simulink model "ServoAmira"  (R2023b)
settings: Solver=ode23  StartTime=0.0  StopTime=10  MaxStep=0.1  RelTol=1e-3  EnableMultiTasking=on
InitFcn:
  | g = 9.81; %gravitational constant
  | 
  | 
  | % showVR = 1; %show VR world
  | % ig_init = 0; %initial condition
  | % im_init = 0; %initial condition
  | % omega_init = 0; %initial condition
  | % phi_init = 0; %initial condition
values from neighbouring files (symbols this model uses):
  b = 2.1E-5    (= 2.1e-05)    [motor_constants.m]
  bg = 1E-5    (= 1e-05)    [motor_constants.m]
  J = 1.8E-5    (= 1.8e-05)    [motor_constants.m]
  Jg = J / 7    (= 2.57142857143e-06)    [motor_constants.m]
  ke = 0.05    [motor_constants.m]
  keg = 0.09    [motor_constants.m]
  km = 0.18    [motor_constants.m]
  kmg = 0.12    [motor_constants.m]
  L = 0.3    [motor_constants.m]
  Lg = 0.1    [motor_constants.m]
  R = 5    [motor_constants.m]
  Rg = 1    [motor_constants.m]
libraries: vrlib x4, slpidlib x2, simulink x1
CloseFcn:
  | vrclose all;
  | clear figureVR worldVR;
settings Model: Creator=Luky  LastModifiedBy=Lenovo
settings DataIOCC: LimitDataPoints=on  SaveFormat=Array  SignalLoggingSaveFormat=ModelDataLogs  ReturnWorkspaceOutputs=off
settings OptimizationCC: ExpressionDepthLimit=2147483647  InitFltsAndDblsToZero=on  LifeSpan=inf
settings DebuggingCC: SaveWithParameterizedLinksMsg=none  UnderspecifiedInitializationDetection=Classic  MergeDetectMultiDrivingBlocksExec=none  SolverPrmCheckMsg=warning  FcnCallInpInsideContextMsg=warning  UnconnectedInputMsg=warning  UnconnectedOutputMsg=warning  UnconnectedLineMsg=warning  StateNameClashWarn=warning  SFUnexpectedBacktrackingDiag=warning  SFNoUnconditionalDefaultTransitionDiag=warning  SFExecutionAtInitializationDiag=none  ArithmeticOperatorsInVariantConditions=warning
settings HardwareCC: ProdBitPerPointer=32  ProdBitPerSizeT=32  ProdBitPerPtrDiffT=32  ProdLargestAtomicFloat=None  ProdIntDivRoundTo=Undefined  ProdEndianess=Unspecified  ProdWordSize=32  ProdHWDeviceType=32-bit Generic
settings ModelReferenceCC: PropagateSignalLabelsOutOfModel=off
settings SFSimCC: SimUseLocalCustomCode=off  CustomCodeUndefinedFunction=UseInterfaceOnly
settings RTWCC: RTWUseLocalCustomCode=off
settings CodeAppCC: StateflowObjectComments=on
settings GRTTargetCC: TargetLangStandard=C89/C90 (ANSI)  CombineOutputUpdateFcns=off  GRTInterface=on
settings ConfigComp: CovMetricSettings=dw  CovSaveCumulativeToWorkspaceVar=on  CovSaveSingleToWorkspaceVar=on  CovExternalEMLEnable=off

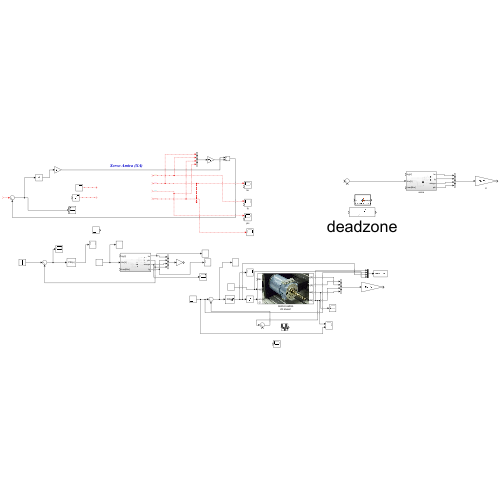
[thumbnail: Simulink's stored preview of the top-level diagram]
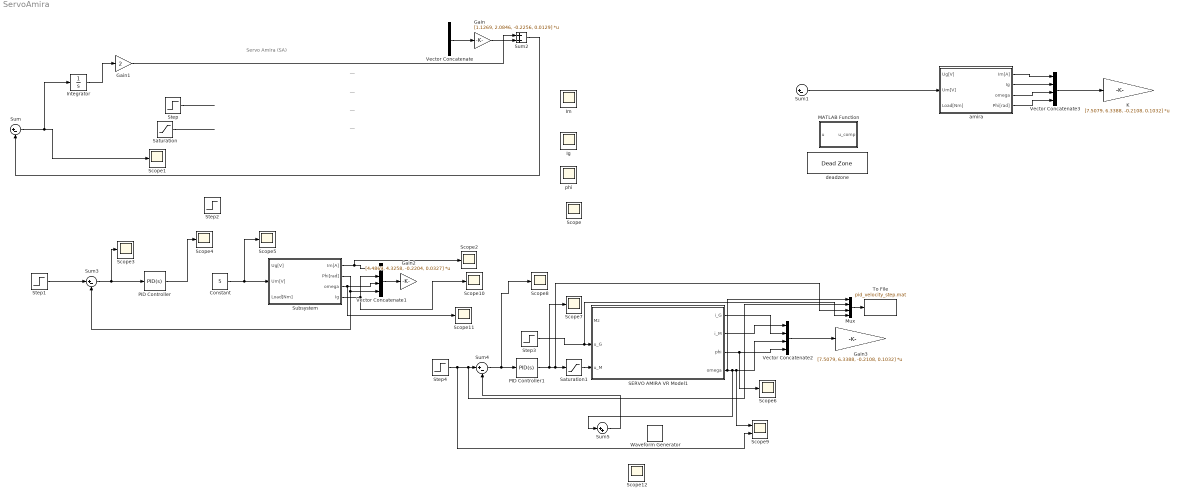
== system ServoAmira ==
  note: Servo Amira (SA)
  note: __
  note: __
  note: __
  note: __
  Constant : Constant  Value=5
  Gain : Gain  Gain=[1.1269, 2.0846, -0.2256, 0.0129]  Multiplication=Matrix(K*u)
  Gain1 : Gain  Gain=2
  Gain2 : Gain  Gain=[4.4869, 4.3258, -0.2204, 0.0327]  Multiplication=Matrix(K*u)
  Gain3 : Gain  Gain=[7.5079, 6.3388, -0.2108, 0.1032]  Multiplication=Matrix(K*u)
  Ig : Scope  NumInputPorts=2
  Im : Scope  NumInputPorts=2
  Integrator : Integrator
  K : Gain  Gain=[7.5079, 6.3388, -0.2108, 0.1032]  Multiplication=Matrix(K*u)
  MATLAB Function : MATLAB Function  TreatAsAtomicUnit=on
  Mux : Mux
  PID Controller : slpidlib/PID Controller  Controller=PID  Form=Parallel  TimeDomain=Continuous-time  UseExternalTs=off  SampleTime=-1  IntegratorMethod=Forward Euler  FilterMethod=Forward Euler  ControllerParametersSource=internal  P=0.1  I=0.1  UseKiTs=off  D=0  N=100  UseFilter=on  TunerSelectOption=Transfer Function Based (PID Tuner App)  InitialConditionSource=internal  InitialConditionForIntegrator=0  InitialConditionForFilter=0  DifferentiatorICPrevScaledInput=0  ExternalReset=none  TrackingMode=off  Kt=1  LimitOutput=off  SatLimitsSource=internal  UpperSaturationLimit=inf  LowerSaturationLimit=-inf  LinearizeAsGain=on  AntiWindupMode=none  Kb=1  LimitIntegrator=off  UpperIntegratorSaturationLimit=inf  LowerIntegratorSaturationLimit=-inf  POutMin=[]  POutMax=[]  IOutMin=[]  IOutMax=[]  DOutMin=[]  DOutMax=[]  NOutMin=[]  NOutMax=[]  SumOutMin=[]  SumOutMax=[]  SaturationOutMin=[]  SaturationOutMax=[]  PParamMin=[]  PParamMax=[]  IParamMin=[]  IParamMax=[]  DParamMin=[]  DParamMax=[]  NParamMin=[]  NParamMax=[]  KbParamMin=[]  KbParamMax=[]  KtParamMin=[]  KtParamMax=[]  KbOutMin=[]  KbOutMax=[]  KtOutMin=[]  KtOutMax=[]  IntegratorOutMin=[]  IntegratorOutMax=[]  FilterOutMin=[]  FilterOutMax=[]  SumI1OutMin=[]  SumI1OutMax=[]  SumI2OutMin=[]  SumI2OutMax=[]  SumI3OutMin=[]  SumI3OutMax=[]  SumI4OutMin=[]  SumI4OutMax=[]  SumDOutMin=[]  SumDOutMax=[]  DifferentiatorOutMin=[]  DifferentiatorOutMax=[]  FilterDiffOutCoefMin=[]  FilterDiffOutCoefMax=[]  ReciprocalOutMin=[]  ReciprocalOutMax=[]  SumDenOutMin=[]  SumDenOutMax=[]  SumNumOutMin=[]  SumNumOutMax=[]  DivideOutMin=[]  DivideOutMax=[]  UdiffTsProdOutMin=[]  UdiffTsProdOutMax=[]  NTsProdOutMin=[]  NTsProdOutMax=[]  UintegralTsProdOutMin=[]  UintegralTsProdOutMax=[]  UngainTsProdOutMin=[]  UngainTsProdOutMax=[]  ClampingZeroOutDataTypeStr=Inherit: Inherit via back propagation  ClampingZeroOutMin=[]  ClampingZeroOutMax=[]  FilterDenConstantOutDataTypeStr=Inherit: Inherit via back propagation  FilterDenConstantOutMin=[]  FilterDenConstantOutMax=[]  PCopyOutDataTypeStr=Inherit: Inherit via back propagation  PCopyOutMin=[]  PCopyOutMax=[]  NCopyOutDataTypeStr=Inherit: Inherit via back propagation  NCopyOutMin=[]  NCopyOutMax=[]  IntegratorContinuousStateAttributes=''  IntegratorStateMustResolveToSignalObject=off  IntegratorRTWStateStorageClass=Auto  FilterContinuousStateAttributes=''  FilterStateMustResolveToSignalObject=off  FilterRTWStateStorageClass=Auto  ParallelPVariant=InternalParameters  IdealPVariant=Disabled  IVariant=InternalParameters  DVariant=InternalParameters  IntegratorVariant=Continuous  SatVariant=Disabled  AWVariant=Passthrough  PCopyVariant=Disabled  TRVariant=Disabled  FdbkBlocksVariant=Forward  IdealPFdbkVariant=Disabled  SatFdbkVariant=Disabled  DerivativeFilterVariant=ContFilter  NVariant=InternalParameters  NCopyVariant=Disabled  FilterICVariant=InternalICsFilter  IntegratorICVariant=InternalICs  ExternalResetVariant=Disabled  TRSumVariant=Passthrough  SumFdbkVariant=Disabled  SumVariant=Sum_PID  TsampFilterVariant=InternalTs  TsampNgainVariant=Passthrough  TsampIntegralVariant=Disabled_SignalSpec  ExternalSaturationOutDataTypeStr=Inherit: Same as second input
  PID Controller1 : slpidlib/PID Controller  Controller=PID  Form=Parallel  TimeDomain=Continuous-time  UseExternalTs=off  SampleTime=-1  IntegratorMethod=Forward Euler  FilterMethod=Forward Euler  ControllerParametersSource=internal  P=0.7401  I=2.6831  UseKiTs=off  D=0.0462  N=150  UseFilter=on  TunerSelectOption=Transfer Function Based (PID Tuner App)  InitialConditionSource=internal  InitialConditionForIntegrator=0  InitialConditionForFilter=0  DifferentiatorICPrevScaledInput=0  ExternalReset=none  TrackingMode=off  Kt=1  LimitOutput=on  SatLimitsSource=internal  UpperSaturationLimit=10  LowerSaturationLimit=-9.9  LinearizeAsGain=on  AntiWindupMode=back-calculation  Kb=1  LimitIntegrator=off  UpperIntegratorSaturationLimit=inf  LowerIntegratorSaturationLimit=-inf  POutMin=[]  POutMax=[]  IOutMin=[]  IOutMax=[]  DOutMin=[]  DOutMax=[]  NOutMin=[]  NOutMax=[]  SumOutMin=[]  SumOutMax=[]  SaturationOutMin=[]  SaturationOutMax=[]  PParamMin=[]  PParamMax=[]  IParamMin=[]  IParamMax=[]  DParamMin=[]  DParamMax=[]  NParamMin=[]  NParamMax=[]  KbParamMin=[]  KbParamMax=[]  KtParamMin=[]  KtParamMax=[]  KbOutMin=[]  KbOutMax=[]  KtOutMin=[]  KtOutMax=[]  IntegratorOutMin=[]  IntegratorOutMax=[]  FilterOutMin=[]  FilterOutMax=[]  SumI1OutMin=[]  SumI1OutMax=[]  SumI2OutMin=[]  SumI2OutMax=[]  SumI3OutMin=[]  SumI3OutMax=[]  SumI4OutMin=[]  SumI4OutMax=[]  SumDOutMin=[]  SumDOutMax=[]  DifferentiatorOutMin=[]  DifferentiatorOutMax=[]  FilterDiffOutCoefMin=[]  FilterDiffOutCoefMax=[]  ReciprocalOutMin=[]  ReciprocalOutMax=[]  SumDenOutMin=[]  SumDenOutMax=[]  SumNumOutMin=[]  SumNumOutMax=[]  DivideOutMin=[]  DivideOutMax=[]  UdiffTsProdOutMin=[]  UdiffTsProdOutMax=[]  NTsProdOutMin=[]  NTsProdOutMax=[]  UintegralTsProdOutMin=[]  UintegralTsProdOutMax=[]  UngainTsProdOutMin=[]  UngainTsProdOutMax=[]  ClampingZeroOutDataTypeStr=Inherit: Inherit via back propagation  ClampingZeroOutMin=[]  ClampingZeroOutMax=[]  FilterDenConstantOutDataTypeStr=Inherit: Inherit via back propagation  FilterDenConstantOutMin=[]  FilterDenConstantOutMax=[]  PCopyOutDataTypeStr=Inherit: Inherit via back propagation  PCopyOutMin=[]  PCopyOutMax=[]  NCopyOutDataTypeStr=Inherit: Inherit via back propagation  NCopyOutMin=[]  NCopyOutMax=[]  IntegratorContinuousStateAttributes=''  IntegratorStateMustResolveToSignalObject=off  IntegratorRTWStateStorageClass=Auto  FilterContinuousStateAttributes=''  FilterStateMustResolveToSignalObject=off  FilterRTWStateStorageClass=Auto  ParallelPVariant=InternalParameters  IdealPVariant=Disabled  IVariant=InternalParameters  DVariant=InternalParameters  IntegratorVariant=Continuous  SatVariant=Enabled  AWVariant=BackCalculation  PCopyVariant=Disabled  TRVariant=Disabled  FdbkBlocksVariant=Forward  IdealPFdbkVariant=Disabled  SatFdbkVariant=Disabled  DerivativeFilterVariant=ContFilter  NVariant=InternalParameters  NCopyVariant=Disabled  FilterICVariant=InternalICsFilter  IntegratorICVariant=InternalICs  ExternalResetVariant=Disabled  TRSumVariant=Passthrough  SumFdbkVariant=Disabled  SumVariant=Sum_PID  TsampFilterVariant=InternalTs  TsampNgainVariant=Passthrough  TsampIntegralVariant=Disabled_SignalSpec  ExternalSaturationOutDataTypeStr=Inherit: Same as second input
  SERVO AMIRA VR Model1 : Subsystem  mask(Servo Amira){showVR=on, sfcnParam1=0, sfcnParam2=0, sfcnParam3=0, sfcnParam4=0}
      mask prompts: showVR "Show VR?"; sfcnParam1 "Initial value of the current of the generator [A]"; sfcnParam2 "Initial value of the current of the motor  im [A]"; sfcnParam3 "Initial value of the angular speed  omega [rad/s]"; sfcnParam4 "Initial value of the angle of the motor shaft phi [rad]"
      mask help: Servo Amira - Virtual Reality
      mask Help:
      | Servo Amira - Virtual Reality <br><br>
      | 
      | 
      | This is a model of the direct current motor. Model is determined to demonstrate real system. It has two inputs, voltage and torgue. Outputs are rotational velocity of the shaft, current and position of the shaft. Virtual reality shows input and output values of the motor.
      | <br><br>
      | 
      | 
      | This is a virtual model of the Servo Amira laboratory model
      | in laboratory of automatic control theory&nbsp;26 (<a href="http://dce.felk.cvut.cz/lab26/" target="_blank">http://dce.felk.cvut.cz/lab26/</a>),
      | which consists of two identical motors (left and right) connected together with a very little flexible shaft. The left motor is used as a generator - it
      | can be used for simulation of a varying  moment of inertia. The right motor is used for control of the rotational speed of the servomechanism or
      | of the angle the motor shaft. <br><br>
      | 
      | There are two inputs and four outputs of the model. The inputs are voltages of the motors um [V] and ug [V] between -10 and 10 volts. Outputs
      | are the speed of the servomechanism omega [rad/s], the angle of the motor shaft phi [rad] and the currents of the motors im [A], ig [A].
      | More information can be found on the website <a href="http://dce.felk.cvut.cz/lab26/" target="_blank">http://dce.felk.cvut.cz/lab26/</a>.<br><br>
      | 
      | 
      | In the mask of the model, it can be set:
      | <ul>
      | <li>Initial value of the current of the generator</li>
      | <li>Initial value of the current of the motor</li>
      | <li>Initial value of the angular speed</li>
      | <li>Initial value of the angle of the motor shaft</li>
      | </ul><br><br>
      | 
      | 
      | Copyright: 2008,   Petr Prochazka, Jirka Roubal, Petr Husek.
      mask Callback showVR:
      | if strcmp('off',get_param(gcb,'showVR'))
      |     vrclose all;
      | else
      |     if exist('figureVR')==0
      |         figureVR = vrfigure;
      |     end
      |     if exist('worldVR')==0
      |         worldVR = vrworld('ServoAmira_VR.WRL');
      |     end
      | 	if isvalid(figureVR)==0
      |         open(worldVR);
      |         figureVR = vrfigure(worldVR,[650 80 550 350]);
      | 	end
      | end
      mask Display:
      | image(imread('ServoAmira_Image.jpg'))
      | port_label ('input',1,'Mz [Nm]')
      | port_label ('input',2,'ug [V]')
      | port_label ('input',3,'um [V]')
      | port_label ('output',1,'ig [A]')
      | port_label ('output',2,'im [A]')
      | port_label ('output',3,'phi [rad]')
      | port_label ('output',4,'omega [rad/s]')
  Saturation : Saturate  UpperLimit=10  LowerLimit=-9.9
  Saturation1 : Saturate  UpperLimit=10  LowerLimit=-9.9
  Scope{,2..8,10..12} (11 alike) : Scope
  Scope1 : Scope  NumInputPorts=3
  Scope9 : Scope  NumInputPorts=2
  Step : Step  Time=2  After=0  SampleTime=0
  Step1 : Step  After=10  SampleTime=0
  Step2 : Step  Time=3  After=0.1  SampleTime=0
  Step3 : Step  Time=4  After=2  SampleTime=0
  Step4 : Step  Time=0  After=20  SampleTime=0
  Subsystem : Subsystem
  Sum{,1,3..4} (4 alike) : Sum  Inputs=|+-
  Sum2 : Sum
  Sum5 : Sum  Inputs=|++
  To File : ToFile  Filename=pid_velocity_step.mat  SaveFormat=Timeseries
  Vector Concatenate{,1..3} (4 alike) : Concatenate  NumInputs=4
  Waveform Generator : simulink/Sources/Waveform Generator  OutMin=[]  OutMax=[]  OutDataTypeStr=double  SelectedSignal=1  Signals=gaussian(0, 0.25, 0)#  BlockNames=MultiportSwitch_1928104fab044be#MultiportSwitch_50f1443cd3b243a  SampleTime=0.05
  amira : Subsystem
  deadzone : DeadZone
  phi : Scope  NumInputPorts=2
  wires:
  ? -> Vector Concatenate/1, Im/1
  ? -> Vector Concatenate/2, Ig/1
  ? -> Vector Concatenate/4, phi/1
  ? -> Vector Concatenate/3, Scope/1
  Step/1 -> ?
  Vector Concatenate/1 -> Gain/1
  Saturation/1 -> ?
  Integrator/1 -> Gain1/1
  Gain1/1 -> Sum2/1
  Gain/1 -> Sum2/2
  Sum2/1 -> Sum/2
  Sum/1 -> Scope1/2, Integrator/1
  ? -> Sum/1
  Vector Concatenate1/1 -> Gain2/1
  Subsystem/1(Im[A]) -> Scope2/1, Vector Concatenate1/1
  Subsystem/4(Ig) -> Scope10/1, Vector Concatenate1/2
  Subsystem/3(omega) -> Scope11/1, Vector Concatenate1/3
  Subsystem/2(Phi[rad]) -> Sum3/2, Vector Concatenate1/4
  Constant/1 -> Scope5/1, Subsystem/2(Um[V])
  Step1/1 -> Sum3/1
  Sum3/1 -> PID Controller/1, Scope3/1
  PID Controller/1 -> Scope4/1
  Vector Concatenate2/1 -> Gain3/1
  SERVO AMIRA VR Model1/2("i_M ") -> Vector Concatenate2/1
  SERVO AMIRA VR Model1/1(i_G) -> Vector Concatenate2/2
  SERVO AMIRA VR Model1/3("phi ") -> Scope6/1, Vector Concatenate2/4
  Saturation1/1 -> SERVO AMIRA VR Model1/3(u_M)
  Mux/1 -> To File/1
  Sum4/1 -> PID Controller1/1, Scope8/1
  Vector Concatenate3/1 -> K/1
  amira/1(Im[A]) -> Vector Concatenate3/1
  amira/2(Ig) -> Vector Concatenate3/2
  amira/3(omega) -> Vector Concatenate3/3
  amira/4(Phi[rad]) -> Vector Concatenate3/4
  Sum1/1 -> amira/2(Um[V])
  PID Controller1/1 -> Scope7/1, Mux/3, Saturation1/1
  SERVO AMIRA VR Model1/4("omega ") -> Mux/1, Sum5/1, Scope9/1, Vector Concatenate2/3
  Step3/1 -> Mux/4, SERVO AMIRA VR Model1/2(u_G)
  Step4/1 -> Scope9/2, Mux/2, Sum4/1
  Sum5/1 -> Sum4/2

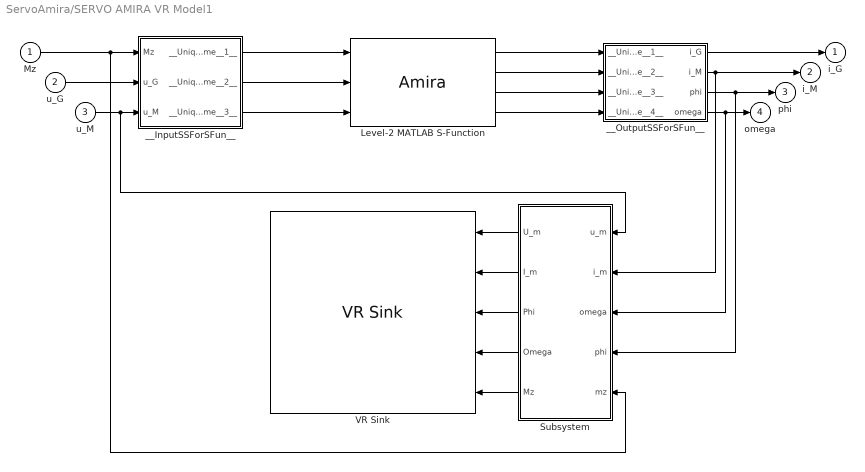
== system ServoAmira/SERVO AMIRA VR Model1 ==
  Mz : Inport
  u_G : Inport  Port=2
  u_M : Inport  Port=3
  Level-2 MATLAB S-Function : M-S-Function  FunctionName=Amira  Parameters=ig0 im0 omega0 psi0  mask{ig0=sfcnParam1, im0=sfcnParam2, omega0=sfcnParam3, psi0=sfcnParam4}
      mask prompts: ig0 "ig_init"; im0 "im_init"; omega0 "omega_init"; psi0 "psi_init"
      mask Display:
      | port_label('input',1,'Mz');
      | port_label('input',2,'u_G');
      | port_label('input',3,'u_M');
      | port_label('output',1,'i_G');
      | port_label('output',2,'i_M ');
      | port_label('output',3,'phi ');
      | port_label('output',4,'omega ');
  Subsystem : Subsystem
  VR Sink : vrlib/VR Sink  InstantiateOnLoad=on  SampleTime=0.1  ViewEnable=on  RemoteChange=off  RemoteView=on  FieldsWritten=show_u.translation.3.1.double#show_i.translation.3.1.double#fi.rotation.4.1.double#show_n.rotation.4.1.double#show_m.translation.3.1.double  WorldFileName=ServoAmira_VR.WRL  AutoView=off  VideoDimensions=[]  AllowVariableSize=off
  __InputSSForSFun__ : Subsystem
  __OutputSSForSFun__ : Subsystem
  i_G : Outport  OutDataTypeStr=double  PortDimensions=1  SampleTime=[-1 0]
  "i_M " : Outport  Port=2  OutDataTypeStr=double  PortDimensions=1  SampleTime=[-1 0]
  "phi " : Outport  Port=3  OutDataTypeStr=double  PortDimensions=1  SampleTime=[-1 0]
  "omega " : Outport  Port=4  OutDataTypeStr=double  PortDimensions=1  SampleTime=[-1 0]
  wires:
  Mz/1 -> __InputSSForSFun__/1(Mz), Subsystem/5(mz)
  u_G/1 -> __InputSSForSFun__/2(u_G)
  u_M/1 -> __InputSSForSFun__/3(u_M), Subsystem/1(u_m)
  __InputSSForSFun__/1(__UniqueOutportName__1__) -> Level-2 MATLAB S-Function/1
  __InputSSForSFun__/2(__UniqueOutportName__2__) -> Level-2 MATLAB S-Function/2
  __InputSSForSFun__/3(__UniqueOutportName__3__) -> Level-2 MATLAB S-Function/3
  Level-2 MATLAB S-Function/1 -> __OutputSSForSFun__/1(__UniqueInportName__1__)
  Level-2 MATLAB S-Function/2 -> __OutputSSForSFun__/2(__UniqueInportName__2__)
  Level-2 MATLAB S-Function/3 -> __OutputSSForSFun__/3(__UniqueInportName__3__)
  Level-2 MATLAB S-Function/4 -> __OutputSSForSFun__/4(__UniqueInportName__4__)
  __OutputSSForSFun__/1(i_G) -> i_G/1
  __OutputSSForSFun__/2("i_M ") -> "i_M "/1, Subsystem/2(i_m)
  __OutputSSForSFun__/3("phi ") -> "phi "/1, Subsystem/4(phi)
  __OutputSSForSFun__/4("omega ") -> "omega "/1, Subsystem/3(omega)
  Subsystem/1(U_m) -> VR Sink/1
  Subsystem/2(I_m) -> VR Sink/2
  Subsystem/5(Mz) -> VR Sink/5
  Subsystem/3(Phi) -> VR Sink/3
  Subsystem/4(Omega) -> VR Sink/4

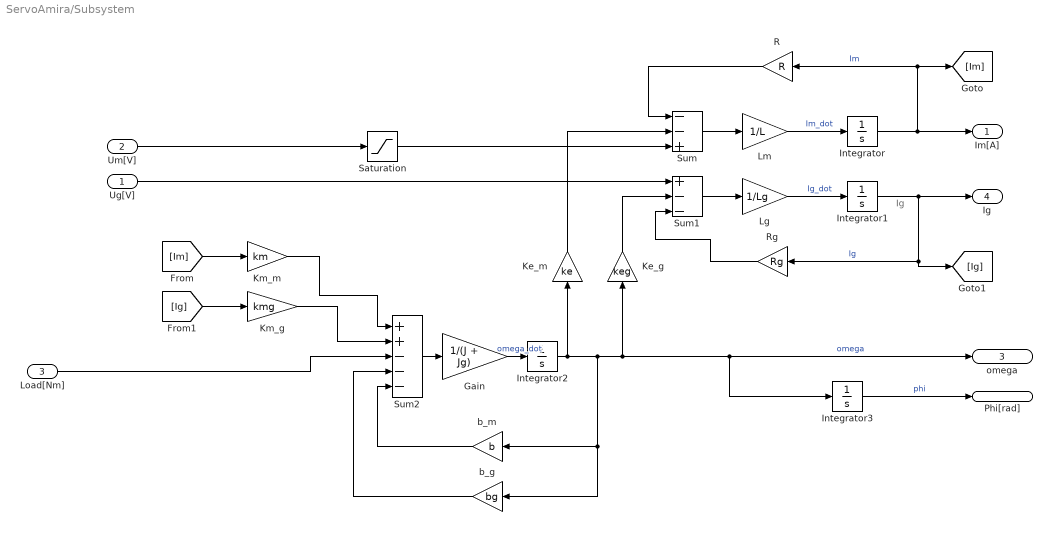
== system ServoAmira/Subsystem ==
  note: Ig
  Ug[V] : Inport
  Um[V] : Inport  Port=2
  Load[Nm] : Inport  Port=3
  Gain : Gain  Gain=1/(J + Jg)
  Integrator{,1..3} (4 alike) : Integrator
  Ke_g : Gain  Gain=keg
  Ke_m : Gain  Gain=ke
  Km_g : Gain  Gain=kmg
  Km_m : Gain  Gain=km
  Lg : Gain  Gain=1/Lg
  Lm : Gain  Gain=1/L
  R : Gain  Gain=R
  Rg : Gain  Gain=Rg
  Saturation : Saturate  UpperLimit=10  LowerLimit=-10
  Sum : Sum  Inputs=--+
  Sum1 : Sum  Inputs=+--
  Sum2 : Sum  Inputs=++---
  b_g : Gain  Gain=bg
  b_m : Gain  Gain=b
  Im[A] : Outport
  Phi[rad] : Outport  Port=2
  omega : Outport  Port=3
  Ig : Outport  Port=4
  wires:
  Integrator/1 -> Im[A]/1, [Im], R/1  "Im"
  [Im] -> Km_m/1
  Lm/1 -> Integrator/1  "Im_dot"
  Integrator2/1 -> omega/1, Integrator3/1, Ke_g/1, b_g/1, b_m/1, Ke_m/1  "omega"
  [Ig] -> Km_g/1
  Km_m/1 -> Sum2/1
  Integrator1/1 -> Ig/1, [Ig], Rg/1  "Ig"
  Sum2/1 -> Gain/1
  Sum/1 -> Lm/1
  Rg/1 -> Sum1/3
  R/1 -> Sum/1
  Ug[V]/1 -> Sum1/1
  Ke_m/1 -> Sum/2
  b_m/1 -> Sum2/5
  Ke_g/1 -> Sum1/2
  Lg/1 -> Integrator1/1  "Ig_dot"
  Sum1/1 -> Lg/1
  b_g/1 -> Sum2/4
  Gain/1 -> Integrator2/1  "omega_dot"
  Integrator3/1 -> Phi[rad]/1  "phi"
  Load[Nm]/1 -> Sum2/3
  Km_g/1 -> Sum2/2
  Um[V]/1 -> Saturation/1
  Saturation/1 -> Sum/3

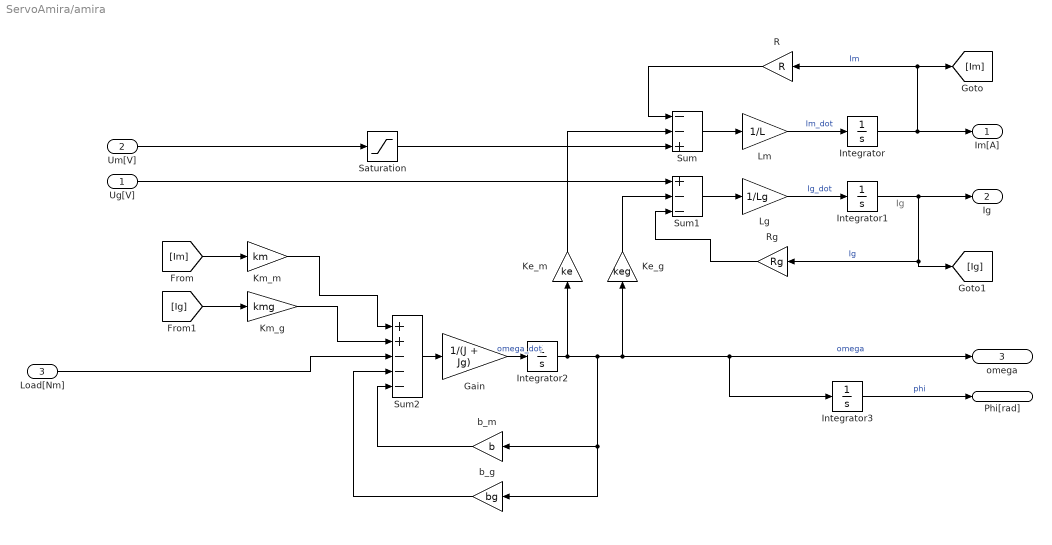
== system ServoAmira/amira ==
  note: Ig
  Ug[V] : Inport
  Um[V] : Inport  Port=2
  Load[Nm] : Inport  Port=3
  Gain : Gain  Gain=1/(J + Jg)
  Integrator{,1..3} (4 alike) : Integrator
  Ke_g : Gain  Gain=keg
  Ke_m : Gain  Gain=ke
  Km_g : Gain  Gain=kmg
  Km_m : Gain  Gain=km
  Lg : Gain  Gain=1/Lg
  Lm : Gain  Gain=1/L
  R : Gain  Gain=R
  Rg : Gain  Gain=Rg
  Saturation : Saturate  UpperLimit=10  LowerLimit=-10
  Sum : Sum  Inputs=--+
  Sum1 : Sum  Inputs=+--
  Sum2 : Sum  Inputs=++---
  b_g : Gain  Gain=bg
  b_m : Gain  Gain=b
  Im[A] : Outport
  Ig : Outport  Port=2
  omega : Outport  Port=3
  Phi[rad] : Outport  Port=4
  wires:
  Integrator/1 -> Im[A]/1, [Im], R/1  "Im"
  [Im] -> Km_m/1
  Lm/1 -> Integrator/1  "Im_dot"
  Integrator2/1 -> omega/1, Integrator3/1, Ke_g/1, b_g/1, b_m/1, Ke_m/1  "omega"
  [Ig] -> Km_g/1
  Km_m/1 -> Sum2/1
  Integrator1/1 -> Ig/1, [Ig], Rg/1  "Ig"
  Sum2/1 -> Gain/1
  Sum/1 -> Lm/1
  Rg/1 -> Sum1/3
  R/1 -> Sum/1
  Ug[V]/1 -> Sum1/1
  Ke_m/1 -> Sum/2
  b_m/1 -> Sum2/5
  Ke_g/1 -> Sum1/2
  Lg/1 -> Integrator1/1  "Ig_dot"
  Sum1/1 -> Lg/1
  b_g/1 -> Sum2/4
  Gain/1 -> Integrator2/1  "omega_dot"
  Integrator3/1 -> Phi[rad]/1  "phi"
  Load[Nm]/1 -> Sum2/3
  Km_g/1 -> Sum2/2
  Um[V]/1 -> Saturation/1
  Saturation/1 -> Sum/3

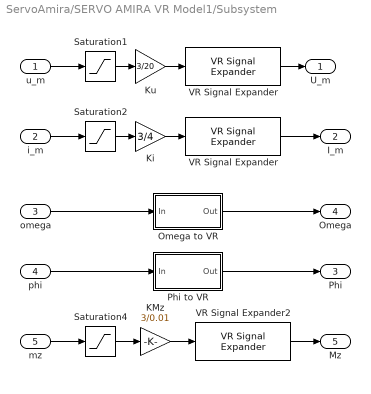
== system ServoAmira/SERVO AMIRA VR Model1/Subsystem ==
  u_m : Inport
  i_m : Inport  Port=2
  omega : Inport  Port=3
  phi : Inport  Port=4
  mz : Inport  Port=5
  KMz : Gain  Gain=3/0.01
  Ki : Gain  Gain=3/4
  Ku : Gain  Gain=3/20
  Omega to VR : Subsystem
  Phi to VR : Subsystem
  Saturation1 : Saturate  UpperLimit=10  LowerLimit=-10
  Saturation2 : Saturate  UpperLimit=4  LowerLimit=-4
  Saturation4 : Saturate  UpperLimit=0.005  LowerLimit=-0.005
  VR Signal Expander : vrlib/VR Signal Expander  outwidth=3  outidx=[2]
  "VR Signal Expander " : vrlib/VR Signal Expander  outwidth=3  outidx=[2]
  VR Signal Expander2 : vrlib/VR Signal Expander  outwidth=3  outidx=[2]
  U_m : Outport
  I_m : Outport  Port=2
  Phi : Outport  Port=3
  Omega : Outport  Port=4
  Mz : Outport  Port=5
  wires:
  Ku/1 -> VR Signal Expander/1
  Saturation1/1 -> Ku/1
  Ki/1 -> "VR Signal Expander "/1
  Saturation2/1 -> Ki/1
  Saturation4/1 -> KMz/1
  KMz/1 -> VR Signal Expander2/1
  u_m/1 -> Saturation1/1
  i_m/1 -> Saturation2/1
  phi/1 -> Phi to VR/1(In)
  omega/1 -> Omega to VR/1(In)
  mz/1 -> Saturation4/1
  VR Signal Expander/1 -> U_m/1
  "VR Signal Expander "/1 -> I_m/1
  Phi to VR/1(Out) -> Phi/1
  Omega to VR/1(Out) -> Omega/1
  VR Signal Expander2/1 -> Mz/1

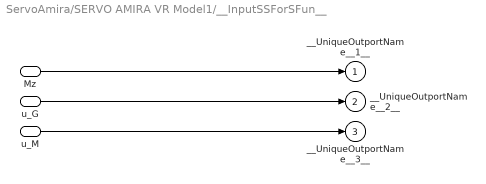
== system ServoAmira/SERVO AMIRA VR Model1/__InputSSForSFun__ ==
  Mz : Inport
  u_G : Inport  Port=2
  u_M : Inport  Port=3
  __UniqueOutportName__1__ : Outport
  __UniqueOutportName__2__ : Outport  Port=2
  __UniqueOutportName__3__ : Outport  Port=3
  wires:
  Mz/1 -> __UniqueOutportName__1__/1
  u_G/1 -> __UniqueOutportName__2__/1
  u_M/1 -> __UniqueOutportName__3__/1

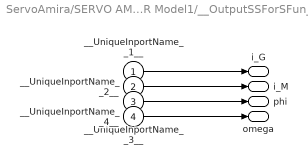
== system ServoAmira/SERVO AMIRA VR Model1/__OutputSSForSFun__ ==
  __UniqueInportName__1__ : Inport
  __UniqueInportName__2__ : Inport  Port=2
  __UniqueInportName__3__ : Inport  Port=3
  __UniqueInportName__4__ : Inport  Port=4
  i_G : Outport  OutDataTypeStr=double  PortDimensions=1  SampleTime=[-1 0]
  "i_M " : Outport  Port=2  OutDataTypeStr=double  PortDimensions=1  SampleTime=[-1 0]
  "phi " : Outport  Port=3  OutDataTypeStr=double  PortDimensions=1  SampleTime=[-1 0]
  "omega " : Outport  Port=4  OutDataTypeStr=double  PortDimensions=1  SampleTime=[-1 0]
  wires:
  __UniqueInportName__1__/1 -> i_G/1
  __UniqueInportName__2__/1 -> "i_M "/1
  __UniqueInportName__3__/1 -> "phi "/1
  __UniqueInportName__4__/1 -> "omega "/1

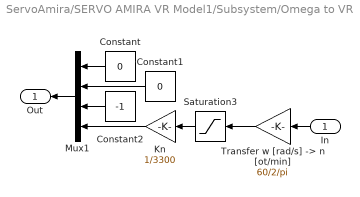
== system ServoAmira/SERVO AMIRA VR Model1/Subsystem/Omega to VR ==
  In : Inport
  Constant : Constant  Value=0
  Constant1 : Constant  Value=0
  Constant2 : Constant  Value=-1
  Kn : Gain  Gain=1/3300
  Mux1 : Mux
  Saturation3 : Saturate  UpperLimit=4500  LowerLimit=-4500
  "Transfer w [rad/s] -> n [ot/min]" : Gain  Gain=60/2/pi
  Out : Outport
  wires:
  Constant/1 -> Mux1/1
  Constant1/1 -> Mux1/2
  Constant2/1 -> Mux1/3
  Saturation3/1 -> Kn/1
  Kn/1 -> Mux1/4
  "Transfer w [rad/s] -> n [ot/min]"/1 -> Saturation3/1
  In/1 -> "Transfer w [rad/s] -> n [ot/min]"/1
  Mux1/1 -> Out/1

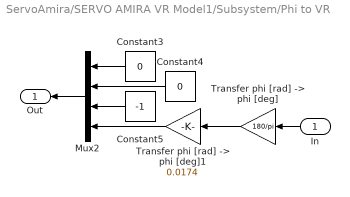
== system ServoAmira/SERVO AMIRA VR Model1/Subsystem/Phi to VR ==
  In : Inport
  Constant3 : Constant  Value=0
  Constant4 : Constant  Value=0
  Constant5 : Constant  Value=-1
  Mux2 : Mux
  "Transfer phi [rad] -> phi [deg]" : Gain  Gain=180/pi
  "Transfer phi [rad] -> phi [deg]1" : Gain  Gain=0.0174
  Out : Outport
  wires:
  Constant3/1 -> Mux2/1
  Constant4/1 -> Mux2/2
  Constant5/1 -> Mux2/3
  In/1 -> "Transfer phi [rad] -> phi [deg]"/1
  Mux2/1 -> Out/1
  "Transfer phi [rad] -> phi [deg]"/1 -> "Transfer phi [rad] -> phi [deg]1"/1
  "Transfer phi [rad] -> phi [deg]1"/1 -> Mux2/4

== matlab function ServoAmira/MATLAB Function ==
  data: u input; u_comp output
function u_comp = deadzone_comp(u)
%#codegen

d = 0.8;  % Deadzone value

if u > 0
    u_comp = u + d;
elseif u < 0
    u_comp = u - d;
else
    u_comp = 0;
end
